simulink model "SimCodeGen_mfun_model"  (R2023b)
settings: Solver=FixedStepAuto  StartTime=0.0  StopTime=10.0  FixedStep=1e-3  RelTol=1e-3
undefined symbols (not defined in the file or in its folder): K, params, x1_ic
settings Model: Creator=Flo  LastModifiedBy=Flo

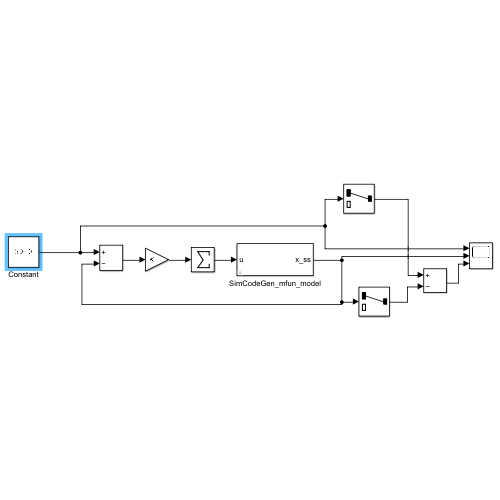
[thumbnail: Simulink's stored preview of the top-level diagram]
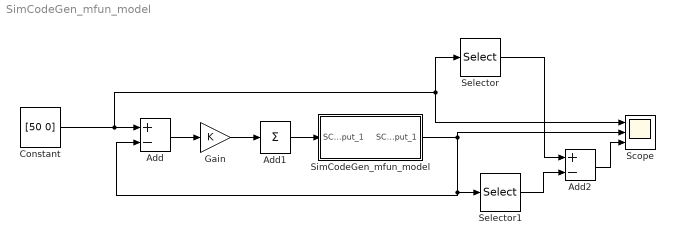
== system SimCodeGen_mfun_model ==
  Add : Sum  Inputs=+-
  Add1 : Sum  Inputs=+
  Add2 : Sum  Inputs=+-
  Constant : Constant  Value=[50 0]  VectorParams1D=off  SampleTime=-1
  Gain : Gain  Gain=K
  Scope : Scope  NumInputPorts=3
  Selector : Selector  InputPortWidth=2  IndexOptions=Index vector (dialog)  Indices=[1]  OutputSizes=1
  Selector1 : Selector  InputPortWidth=2  IndexOptions=Index vector (dialog)  Indices=[1]  OutputSizes=1
  SimCodeGen_mfun_model : Subsystem  mask{SC_param_0=params, SC_x1_ic=x1_ic}
      mask prompts: SC_param_0 "params"
      mask Display:
      | port_label('input', 1, 'u');
      | port_label('output', 1, 'x_ss');
  wires:
  SimCodeGen_mfun_model/1(SC_output_1) -> Add/2, Selector1/1, Scope/2
  Add1/1 -> SimCodeGen_mfun_model/1(SC_input_1)
  Gain/1 -> Add1/1
  Add/1 -> Gain/1
  Constant/1 -> Selector/1, Scope/1, Add/1
  Selector/1 -> Add2/1
  Selector1/1 -> Add2/2
  Add2/1 -> Scope/3

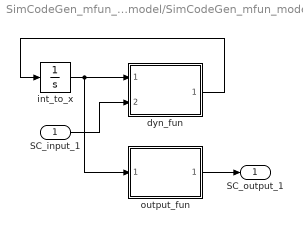
== system SimCodeGen_mfun_model/SimCodeGen_mfun_model ==
  SC_input_1 : Inport
  dyn_fun : MATLAB Function  TreatAsAtomicUnit=on
  int_to_x : Integrator  InitialCondition=[SC_x1_ic]
  output_fun : MATLAB Function  TreatAsAtomicUnit=on
  SC_output_1 : Outport
  wires:
  dyn_fun/1(SC_state_dot) -> int_to_x/1
  int_to_x/1 -> dyn_fun/1(SC_state), output_fun/1(SC_state)
  SC_input_1/1 -> dyn_fun/2(SC_input_0)
  output_fun/1(SC_output_0) -> SC_output_1/1

== matlab function SimCodeGen_mfun_model/dyn_fun ==
  data: SC_state input size=[2]; SC_state_dot output size=[2]; SC_input_0 input size=[1]; SC_param_0 parameter
function SC_state_dot  = dyn_fun(SC_state, SC_input_0, SC_param_0)
    SC_state_dot = zeros(2, 1);
    SC_state_x_0 = SC_state(1:2);
    SC_eval = zeros(2,1);
    SC_eval(1) = SC_state_x_0(2);
    t1 = SC_param_0(1);
    t5 = conj(SC_param_0(4) * t1);
    SC_eval(2) = -(SC_eval(1) * SC_param_0(3) + SC_param_0(2) * SC_state_x_0(1) - t5 - SC_input_0(1)) / t1;
    SC_state_dot(1:2) = SC_eval(1:2);
end

== matlab function SimCodeGen_mfun_model/output_fun ==
  data: SC_state input size=[2]; SC_output_0 output size=[2]; SC_param_0 parameter size=[4]
function SC_output_0  = y_fun(SC_state, SC_param_0)
    SC_output_0 = zeros(2,1);
    SC_state_x_0 = SC_state(1:2);
    SC_output_0(1) = SC_state_x_0(1);
    SC_output_0(2) = SC_state_x_0(2);
end
